simulink subsystem "April_Tag_Relative_Errors"  (R2023b)
settings: Solver=VariableStepAuto  StartTime=0.0  StopTime=10.0  RelTol=1e-3
undefined symbols (not defined in the file): AT_Integral_Enable_Error_Angle, AT_Integral_Enable_Error_XY, AT_Max_Error_Angle, AT_Max_Error_XY, AT_Reef_Target_Algae_X, AT_Reef_Target_Algae_Y, AT_Reef_Target_Center_Y, AT_Reef_Target_L1_X, AT_Reef_Target_L2_L3_X, AT_Reef_Target_L4_X, AT_Reef_Target_Left_Y, AT_Reef_Target_Right_Y
libraries: simulink x18
settings Model: Creator=ander  LastModifiedBy=ander

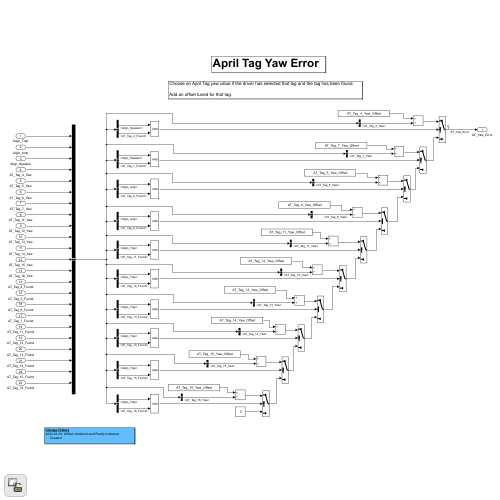
[thumbnail: Simulink's stored preview of the top-level diagram]
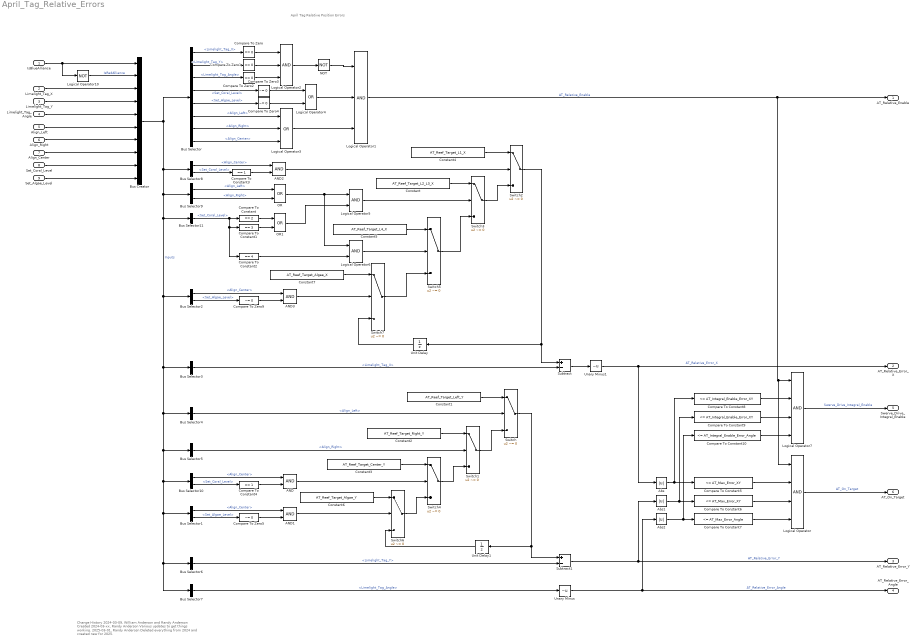
== system April_Tag_Relative_Errors ==
  note: Change History
      | 2024-03-09, William Anderson and Randy Anderson
      | Created
      | 2024-03-xx, Randy Anderson
      | Various updates to get things working.
      | 2025-03-01, Randy Anderosn
      | Deleted everything from 2024 and created new for 2025.
  note: April Tag Relative Position Errors
  IsBlueAlliance : Inport
  Limelight_Tag_X : Inport  Port=2
  Limelight_Tag_Y : Inport  Port=3
  Limelight_Tag_Angle : Inport  Port=4
  Align_Left : Inport  Port=5
  Align_Right : Inport  Port=6
  Align_Center : Inport  Port=7
  Set_Coral_Level : Inport  Port=8
  Set_Algae_Level : Inport  Port=9
  AND{,1..3} (4 alike) : Logic  AllPortsSameDT=off  OutDataTypeStr=boolean
  Abs : Abs  SaturateOnIntegerOverflow=off
  Abs1 : Abs  SaturateOnIntegerOverflow=off
  Abs2 : Abs  SaturateOnIntegerOverflow=off
  Bus Creator : BusCreator  Inputs=10
  Bus Selector : BusSelector  OutputSignals=Limelight_Tag_X,Limelight_Tag_Y,Limelight_Tag_Angle,Set_Coral_Level,Set_Algae_Level,Align_Left,Align_Right,Align_Center
  Bus Selector1 : BusSelector  OutputSignals=Align_Center,Set_Algae_Level
  Bus Selector10 : BusSelector  OutputSignals=Align_Center,Set_Coral_Level
  Bus Selector11 : BusSelector  OutputSignals=Set_Coral_Level
  Bus Selector2 : BusSelector  OutputSignals=Align_Center,Set_Algae_Level
  Bus Selector3 : BusSelector  OutputSignals=Limelight_Tag_X
  Bus Selector4 : BusSelector  OutputSignals=Align_Left
  Bus Selector5 : BusSelector  OutputSignals=Align_Right
  Bus Selector6 : BusSelector  OutputSignals=Limelight_Tag_Y
  Bus Selector7 : BusSelector  OutputSignals=Limelight_Tag_Angle
  Bus Selector8 : BusSelector  OutputSignals=Align_Center,Set_Coral_Level
  Bus Selector9 : BusSelector  OutputSignals=Align_Left,Align_Right
  Compare To Constant : simulink/Logic and Bit Operations/Compare To Constant  relop===  const=2  OutDataTypeStr=boolean
  Compare To Constant1 : simulink/Logic and Bit Operations/Compare To Constant  relop===  const=3  OutDataTypeStr=boolean
  Compare To Constant10 : simulink/Logic and Bit Operations/Compare To Constant  relop=<=  const=AT_Integral_Enable_Error_Angle  OutDataTypeStr=boolean
  Compare To Constant2 : simulink/Logic and Bit Operations/Compare To Constant  relop===  const=4  OutDataTypeStr=boolean
  Compare To Constant3 : simulink/Logic and Bit Operations/Compare To Constant  relop===  const=1  OutDataTypeStr=boolean
  Compare To Constant4 : simulink/Logic and Bit Operations/Compare To Constant  relop===  const=1  OutDataTypeStr=boolean
  Compare To Constant5 : simulink/Logic and Bit Operations/Compare To Constant  relop=<=  const=AT_Max_Error_XY  OutDataTypeStr=boolean
  Compare To Constant6 : simulink/Logic and Bit Operations/Compare To Constant  relop=<=  const=AT_Max_Error_XY  OutDataTypeStr=boolean
  Compare To Constant7 : simulink/Logic and Bit Operations/Compare To Constant  relop=<=  const=AT_Max_Error_Angle  OutDataTypeStr=boolean
  Compare To Constant8 : simulink/Logic and Bit Operations/Compare To Constant  relop=<=  const=AT_Integral_Enable_Error_XY  OutDataTypeStr=boolean
  Compare To Constant9 : simulink/Logic and Bit Operations/Compare To Constant  relop=<=  const=AT_Integral_Enable_Error_XY  OutDataTypeStr=boolean
  Compare To Zero : simulink/Logic and Bit Operations/Compare To Zero  relop===  OutDataTypeStr=boolean
  Compare To Zero1 : simulink/Logic and Bit Operations/Compare To Zero  relop===  OutDataTypeStr=boolean
  Compare To Zero2 : simulink/Logic and Bit Operations/Compare To Zero  relop===  OutDataTypeStr=boolean
  Compare To Zero{3..5,9} (4 alike) : simulink/Logic and Bit Operations/Compare To Zero  relop=~=  OutDataTypeStr=boolean
  Constant : Constant  Value=AT_Reef_Target_L2_L3_X
  Constant1 : Constant  Value=AT_Reef_Target_Left_Y
  Constant2 : Constant  Value=AT_Reef_Target_Right_Y
  Constant3 : Constant  Value=AT_Reef_Target_Center_Y
  Constant4 : Constant  Value=AT_Reef_Target_L1_X
  Constant5 : Constant  Value=AT_Reef_Target_L4_X
  Constant6 : Constant  Value=AT_Reef_Target_Algae_Y
  Constant7 : Constant  Value=AT_Reef_Target_Algae_X
  Logical Operator : Logic  Inputs=4  AllPortsSameDT=off  OutDataTypeStr=boolean
  Logical Operator1 : Logic  Inputs=3  AllPortsSameDT=off  OutDataTypeStr=boolean
  Logical Operator10 : Logic  Operator=NOT  AllPortsSameDT=off  OutDataTypeStr=boolean
  Logical Operator2 : Logic  Inputs=3  AllPortsSameDT=off  OutDataTypeStr=boolean
  Logical Operator3 : Logic  Operator=OR  Inputs=3  AllPortsSameDT=off  OutDataTypeStr=boolean
  Logical Operator4 : Logic  Operator=OR  AllPortsSameDT=off  OutDataTypeStr=boolean
  Logical Operator5 : Logic  AllPortsSameDT=off  OutDataTypeStr=boolean
  Logical Operator6 : Logic  AllPortsSameDT=off  OutDataTypeStr=boolean
  Logical Operator7 : Logic  Inputs=4  AllPortsSameDT=off  OutDataTypeStr=boolean
  NOT : Logic  Operator=NOT  AllPortsSameDT=off  OutDataTypeStr=boolean
  OR : Logic  Operator=OR  AllPortsSameDT=off  OutDataTypeStr=boolean
  OR1 : Logic  Operator=OR  AllPortsSameDT=off  OutDataTypeStr=boolean
  Subtract : Sum  Inputs=+-
  Subtract1 : Sum  Inputs=+-
  Switch{,1..7} (8 alike) : Switch  Criteria=u2 ~= 0  SaturateOnIntegerOverflow=off  InputSameDT=off
  Unary Minus : UnaryMinus
  Unary Minus1 : UnaryMinus
  Unit Delay : UnitDelay  SampleTime=-1  HasFrameUpgradeWarning=on
  Unit Delay1 : UnitDelay  SampleTime=-1  HasFrameUpgradeWarning=on
  AT_Relative_Enable : Outport
  AT_Relative_Error_X : Outport  Port=2
  AT_Relative_Error_Y : Outport  Port=3
  AT_Relative_Error_Angle : Outport  Port=4
  Swerve_Drive_Integral_Enable : Outport  Port=5
  AT_On_Target : Outport  Port=6
  wires:
  Align_Center/1 -> Bus Creator/8
  Align_Right/1 -> Bus Creator/7
  Align_Left/1 -> Bus Creator/6
  Limelight_Tag_Angle/1 -> Bus Creator/5
  Limelight_Tag_Y/1 -> Bus Creator/4
  Limelight_Tag_X/1 -> Bus Creator/3
  Set_Coral_Level/1 -> Bus Creator/9
  IsBlueAlliance/1 -> Bus Creator/1, Logical Operator10/1
  Bus Creator/1 -> Bus Selector9/1, Bus Selector11/1, Bus Selector3/1, Bus Selector4/1, Bus Selector10/1, Bus Selector1/1, Bus Selector6/1, Bus Selector7/1, Bus Selector5/1, Bus Selector2/1, Bus Selector8/1, Bus Selector/1  "Inputs"
  Bus Selector/1 -> Compare To Zero/1  "<Limelight_Tag_X>"
  Bus Selector/2 -> Compare To Zero1/1  "<Limelight_Tag_Y>"
  Bus Selector/3 -> Compare To Zero2/1  "<Limelight_Tag_Angle>"
  Compare To Zero/1 -> Logical Operator2/1
  Compare To Zero1/1 -> Logical Operator2/2
  Compare To Zero2/1 -> Logical Operator2/3
  NOT/1 -> Logical Operator1/1
  Logical Operator1/1 -> AT_Relative_Enable/1, Logical Operator7/1, Logical Operator/1  "AT_Relative_Enable"
  Bus Selector3/1 -> Subtract/2  "<Limelight_Tag_X>"
  Constant1/1 -> Switch/1
  Bus Selector4/1 -> Switch/2  "<Align_Left>"
  Switch1/1 -> Switch/3
  Bus Selector5/1 -> Switch1/2  "<Align_Right>"
  Constant2/1 -> Switch1/1
  Switch/1 -> Subtract1/1, Unit Delay1/1
  Bus Selector6/1 -> Subtract1/2  "<Limelight_Tag_Y>"
  Subtract/1 -> Unary Minus1/1
  Subtract1/1 -> AT_Relative_Error_Y/1, Abs1/1  "AT_Relative_Error_Y"
  Bus Selector7/1 -> Unary Minus/1  "<Limelight_Tag_Angle>"
  Unary Minus/1 -> Abs2/1, AT_Relative_Error_Angle/1  "AT_Relative_Error_Angle"
  Unary Minus1/1 -> AT_Relative_Error_X/1, Abs/1  "AT_Relative_Error_X"
  Constant4/1 -> Switch2/1
  Switch2/1 -> Unit Delay/1, Subtract/1
  Switch3/1 -> Switch2/3
  Constant/1 -> Switch3/1
  Bus Selector9/1 -> OR/1  "<Align_Left>"
  Bus Selector9/2 -> OR/2  "<Align_Right>"
  Switch4/1 -> Switch1/3
  Constant3/1 -> Switch4/1
  Unit Delay1/1 -> Switch6/3
  OR/1 -> Logical Operator5/1, Logical Operator6/1
  Switch5/1 -> Switch3/3
  Constant5/1 -> Switch5/1
  Logical Operator6/1 -> Switch5/2
  Logical Operator5/1 -> Switch3/2
  OR1/1 -> Logical Operator5/2
  Compare To Constant/1 -> OR1/1
  Compare To Constant1/1 -> OR1/2
  Compare To Constant2/1 -> Logical Operator6/2
  Logical Operator10/1 -> Bus Creator/2  "IsRedAlliance"
  Bus Selector11/1 -> Compare To Constant/1, Compare To Constant1/1, Compare To Constant2/1  "<Set_Coral_Level>"
  Bus Selector/4 -> Compare To Zero3/1  "<Set_Coral_Level>"
  Logical Operator3/1 -> Logical Operator1/3
  Logical Operator2/1 -> NOT/1
  Bus Selector/6 -> Logical Operator3/1  "<Align_Left>"
  Bus Selector/7 -> Logical Operator3/2  "<Align_Right>"
  Bus Selector/8 -> Logical Operator3/3  "<Align_Center>"
  Set_Algae_Level/1 -> Bus Creator/10
  Bus Selector/5 -> Compare To Zero4/1  "<Set_Algae_Level>"
  Compare To Zero3/1 -> Logical Operator4/1
  Compare To Zero4/1 -> Logical Operator4/2
  Logical Operator4/1 -> Logical Operator1/2
  Bus Selector10/1 -> AND/1  "<Align_Center>"
  Bus Selector10/2 -> Compare To Constant4/1  "<Set_Coral_Level>"
  Bus Selector1/1 -> AND1/1  "<Align_Center>"
  Bus Selector1/2 -> Compare To Zero5/1  "<Set_Algae_Level>"
  Compare To Zero5/1 -> AND1/2
  AND/1 -> Switch4/2
  Switch6/1 -> Switch4/3
  AND1/1 -> Switch6/2
  Constant6/1 -> Switch6/1
  Compare To Constant3/1 -> AND2/2
  Bus Selector8/1 -> AND2/1  "<Align_Center>"
  Bus Selector8/2 -> Compare To Constant3/1  "<Set_Coral_Level>"
  AND2/1 -> Switch2/2
  Switch7/1 -> Switch5/3
  Compare To Zero9/1 -> AND3/2
  Bus Selector2/1 -> AND3/1  "<Align_Center>"
  Bus Selector2/2 -> Compare To Zero9/1  "<Set_Algae_Level>"
  AND3/1 -> Switch7/2
  Constant7/1 -> Switch7/1
  Unit Delay/1 -> Switch7/3
  Compare To Constant4/1 -> AND/2
  Abs/1 -> Compare To Constant5/1, Compare To Constant8/1
  Abs2/1 -> Compare To Constant7/1, Compare To Constant10/1
  Abs1/1 -> Compare To Constant6/1, Compare To Constant9/1
  Logical Operator/1 -> AT_On_Target/1  "AT_On_Target"
  Compare To Constant8/1 -> Logical Operator7/2
  Compare To Constant10/1 -> Logical Operator7/4
  Compare To Constant9/1 -> Logical Operator7/3
  Logical Operator7/1 -> Swerve_Drive_Integral_Enable/1  "Swerve_Drive_Integral_Enable"
  Compare To Constant5/1 -> Logical Operator/2
  Compare To Constant6/1 -> Logical Operator/3
  Compare To Constant7/1 -> Logical Operator/4
